simulink model "PhysicalHyperCook"  (R2026b)
settings: Solver=VariableStepAuto  StopTime=14400
undefined symbols (not defined in the file): Fault_T_Cook1, Fault_T_Cook2, Fault_T_Cook3, Fault_T_Cook4, Fault_T_Pack, Fault_T_Prep1, Fault_T_Prep2, Fault_T_QC, HC_PackRate_bph, HC_PrepRate_bph, HC_QCRate_bph, HC_Resupply_bph, Recipe_Block_s, Recipe_Count, Recipe_Flush_s, Resupply_Cutoff_T, Transport_Latency_s, Transport_Rate_bph
(part 1 of 2)
settings Model: DataDictionary=PhysicalHyperCookData.sldd  Creator=sarah  LastModifiedBy=sdagen

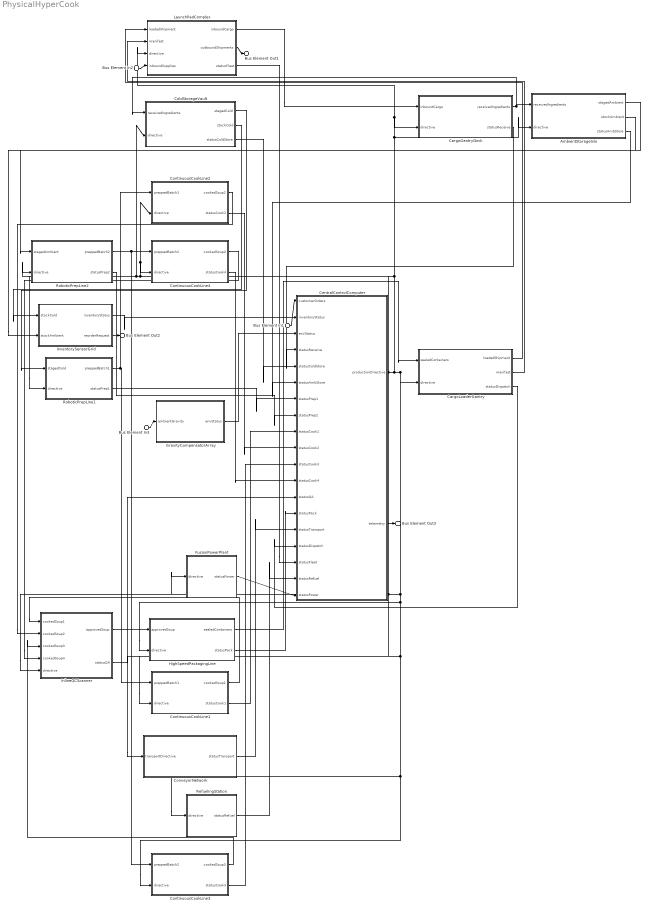
== system PhysicalHyperCook ==
  Bus Element In1 : Inport  PortName=CustomerOrders
  Bus Element In2 : Inport  Port=2  PortName=InboundSupplies
  Bus Element In3 : Inport  Port=3  PortName=AmbientGravity
  AmbientStorageSilo : Subsystem
      settings: PortSchema="{\"entries\":[{\"content\":{\"headerSize\":26,\"margin\":15,\"minimumSpacing\":25,\"sides\":[{\"content\":{\"connectorIds\":[\"In1\",\"In2\"]},\"type\":\"ConnectorPlacement.EquallySpacedRectSide\",\"uuid\":\"f830f98a-8e8b-4468-adf4-d6eab644987f\"},{\"content\":{\"connectorIds\":[\"Out1\",\"Out2\",\"Out3\"],\"side\":\"RIGHT\"},\"type\":\"ConnectorPlacement.EquallySpacedRectSide\",\"uuid\":\"7e0d0116-b3ba-4668-b638-30d0f54ba087\"},{\"content\":{\"side\":\"TOP\"},\"type\":\"ConnectorPlacement.EquallySpacedRectSide\",\"uuid\":\"7b4146d3-46d2-45ca-8c34-b106f0d8cedd\"}]},\"type\":\"ConnectorPlacement.EquallySpacedConnector\",\"uuid\":\"3d911b2d-a78f-42ea-b869-5e09982d9f54\"}],\"packageUris\":[\"http://schema.mathworks.com/mf0/Connector/R2020b\"],\"version\":\"1.0\"}"
  CargoGantryDock : Subsystem
      settings: PortSchema="{\"entries\":[{\"content\":{\"headerSize\":26,\"margin\":15,\"minimumSpacing\":25,\"sides\":[{\"content\":{\"connectorIds\":[\"In1\",\"In2\"]},\"type\":\"ConnectorPlacement.EquallySpacedRectSide\",\"uuid\":\"f830f98a-8e8b-4468-adf4-d6eab644987f\"},{\"content\":{\"connectorIds\":[\"Out1\",\"Out2\"],\"side\":\"RIGHT\"},\"type\":\"ConnectorPlacement.EquallySpacedRectSide\",\"uuid\":\"7e0d0116-b3ba-4668-b638-30d0f54ba087\"},{\"content\":{\"side\":\"TOP\"},\"type\":\"ConnectorPlacement.EquallySpacedRectSide\",\"uuid\":\"7b4146d3-46d2-45ca-8c34-b106f0d8cedd\"}]},\"type\":\"ConnectorPlacement.EquallySpacedConnector\",\"uuid\":\"3d911b2d-a78f-42ea-b869-5e09982d9f54\"}],\"packageUris\":[\"http://schema.mathworks.com/mf0/Connector/R2020b\"],\"version\":\"1.0\"}"
  CargoLoaderGantry : Subsystem
      settings: PortSchema="{\"entries\":[{\"content\":{\"headerSize\":26,\"margin\":15,\"minimumSpacing\":25,\"sides\":[{\"content\":{\"connectorIds\":[\"In1\",\"In2\"]},\"type\":\"ConnectorPlacement.EquallySpacedRectSide\",\"uuid\":\"f830f98a-8e8b-4468-adf4-d6eab644987f\"},{\"content\":{\"connectorIds\":[\"Out1\",\"Out2\",\"Out3\"],\"side\":\"RIGHT\"},\"type\":\"ConnectorPlacement.EquallySpacedRectSide\",\"uuid\":\"7e0d0116-b3ba-4668-b638-30d0f54ba087\"},{\"content\":{\"side\":\"TOP\"},\"type\":\"ConnectorPlacement.EquallySpacedRectSide\",\"uuid\":\"7b4146d3-46d2-45ca-8c34-b106f0d8cedd\"}]},\"type\":\"ConnectorPlacement.EquallySpacedConnector\",\"uuid\":\"3d911b2d-a78f-42ea-b869-5e09982d9f54\"}],\"packageUris\":[\"http://schema.mathworks.com/mf0/Connector/R2020b\"],\"version\":\"1.0\"}"
  CentralControlComputer : Subsystem
      settings: PortSchema="{\"entries\":[{\"content\":{\"headerSize\":26,\"margin\":15,\"minimumSpacing\":25,\"sides\":[{\"content\":{\"connectorIds\":[\"In1\",\"In2\",\"In3\",\"In4\",\"In5\",\"In6\",\"In7\",\"In8\",\"In9\",\"In10\",\"In11\",\"In12\",\"In13\",\"In14\",\"In15\",\"In16\",\"In17\",\"In18\",\"In19\"]},\"type\":\"ConnectorPlacement.EquallySpacedRectSide\",\"uuid\":\"f830f98a-8e8b-4468-adf4-d6eab644987f\"},{\"content\":{\"connectorIds\":[\"Out1\",\"Out2\"],\"side\":\"RIGHT\"},\"type\":\"ConnectorPlacement.EquallySpacedRectSide\",\"uuid\":\"7e0d0116-b3ba-4668-b638-30d0f54ba087\"},{\"content\":{\"side\":\"TOP\"},\"type\":\"ConnectorPlacement.EquallySpacedRectSide\",\"uuid\":\"7b4146d3-46d2-45ca-8c34-b106f0d8cedd\"}]},\"type\":\"ConnectorPlacement.EquallySpacedConnector\",\"uuid\":\"3d911b2d-a78f-42ea-b869-5e09982d9f54\"}],\"packageUris\":[\"http://schema.mathworks.com/mf0/Connector/R2020b\"],\"version\":\"1.0\"}"
  ColdStorageVault : Subsystem
      settings: PortSchema="{\"entries\":[{\"content\":{\"headerSize\":26,\"margin\":15,\"minimumSpacing\":25,\"sides\":[{\"content\":{\"connectorIds\":[\"In1\",\"In2\"]},\"type\":\"ConnectorPlacement.EquallySpacedRectSide\",\"uuid\":\"f830f98a-8e8b-4468-adf4-d6eab644987f\"},{\"content\":{\"connectorIds\":[\"Out1\",\"Out2\",\"Out3\"],\"side\":\"RIGHT\"},\"type\":\"ConnectorPlacement.EquallySpacedRectSide\",\"uuid\":\"7e0d0116-b3ba-4668-b638-30d0f54ba087\"},{\"content\":{\"side\":\"TOP\"},\"type\":\"ConnectorPlacement.EquallySpacedRectSide\",\"uuid\":\"7b4146d3-46d2-45ca-8c34-b106f0d8cedd\"}]},\"type\":\"ConnectorPlacement.EquallySpacedConnector\",\"uuid\":\"3d911b2d-a78f-42ea-b869-5e09982d9f54\"}],\"packageUris\":[\"http://schema.mathworks.com/mf0/Connector/R2020b\"],\"version\":\"1.0\"}"
  ContinuousCookLine1 : Subsystem
      settings: PortSchema="{\"entries\":[{\"content\":{\"headerSize\":26,\"margin\":15,\"minimumSpacing\":25,\"sides\":[{\"content\":{\"connectorIds\":[\"In1\",\"In2\"]},\"type\":\"ConnectorPlacement.EquallySpacedRectSide\",\"uuid\":\"f830f98a-8e8b-4468-adf4-d6eab644987f\"},{\"content\":{\"connectorIds\":[\"Out1\",\"Out2\"],\"side\":\"RIGHT\"},\"type\":\"ConnectorPlacement.EquallySpacedRectSide\",\"uuid\":\"7e0d0116-b3ba-4668-b638-30d0f54ba087\"},{\"content\":{\"side\":\"TOP\"},\"type\":\"ConnectorPlacement.EquallySpacedRectSide\",\"uuid\":\"7b4146d3-46d2-45ca-8c34-b106f0d8cedd\"}]},\"type\":\"ConnectorPlacement.EquallySpacedConnector\",\"uuid\":\"3d911b2d-a78f-42ea-b869-5e09982d9f54\"}],\"packageUris\":[\"http://schema.mathworks.com/mf0/Connector/R2020b\"],\"version\":\"1.0\"}"
  ContinuousCookLine2 : Subsystem
      settings: PortSchema="{\"entries\":[{\"content\":{\"headerSize\":26,\"margin\":15,\"minimumSpacing\":25,\"sides\":[{\"content\":{\"connectorIds\":[\"In1\",\"In2\"]},\"type\":\"ConnectorPlacement.EquallySpacedRectSide\",\"uuid\":\"f830f98a-8e8b-4468-adf4-d6eab644987f\"},{\"content\":{\"connectorIds\":[\"Out1\",\"Out2\"],\"side\":\"RIGHT\"},\"type\":\"ConnectorPlacement.EquallySpacedRectSide\",\"uuid\":\"7e0d0116-b3ba-4668-b638-30d0f54ba087\"},{\"content\":{\"side\":\"TOP\"},\"type\":\"ConnectorPlacement.EquallySpacedRectSide\",\"uuid\":\"7b4146d3-46d2-45ca-8c34-b106f0d8cedd\"}]},\"type\":\"ConnectorPlacement.EquallySpacedConnector\",\"uuid\":\"3d911b2d-a78f-42ea-b869-5e09982d9f54\"}],\"packageUris\":[\"http://schema.mathworks.com/mf0/Connector/R2020b\"],\"version\":\"1.0\"}"
  ContinuousCookLine3 : Subsystem
      settings: PortSchema="{\"entries\":[{\"content\":{\"headerSize\":26,\"margin\":15,\"minimumSpacing\":25,\"sides\":[{\"content\":{\"connectorIds\":[\"In1\",\"In2\"]},\"type\":\"ConnectorPlacement.EquallySpacedRectSide\",\"uuid\":\"f830f98a-8e8b-4468-adf4-d6eab644987f\"},{\"content\":{\"connectorIds\":[\"Out1\",\"Out2\"],\"side\":\"RIGHT\"},\"type\":\"ConnectorPlacement.EquallySpacedRectSide\",\"uuid\":\"7e0d0116-b3ba-4668-b638-30d0f54ba087\"},{\"content\":{\"side\":\"TOP\"},\"type\":\"ConnectorPlacement.EquallySpacedRectSide\",\"uuid\":\"7b4146d3-46d2-45ca-8c34-b106f0d8cedd\"}]},\"type\":\"ConnectorPlacement.EquallySpacedConnector\",\"uuid\":\"3d911b2d-a78f-42ea-b869-5e09982d9f54\"}],\"packageUris\":[\"http://schema.mathworks.com/mf0/Connector/R2020b\"],\"version\":\"1.0\"}"
  ContinuousCookLine4 : Subsystem
      settings: PortSchema="{\"entries\":[{\"content\":{\"headerSize\":26,\"margin\":15,\"minimumSpacing\":25,\"sides\":[{\"content\":{\"connectorIds\":[\"In1\",\"In2\"]},\"type\":\"ConnectorPlacement.EquallySpacedRectSide\",\"uuid\":\"f830f98a-8e8b-4468-adf4-d6eab644987f\"},{\"content\":{\"connectorIds\":[\"Out1\",\"Out2\"],\"side\":\"RIGHT\"},\"type\":\"ConnectorPlacement.EquallySpacedRectSide\",\"uuid\":\"7e0d0116-b3ba-4668-b638-30d0f54ba087\"},{\"content\":{\"side\":\"TOP\"},\"type\":\"ConnectorPlacement.EquallySpacedRectSide\",\"uuid\":\"7b4146d3-46d2-45ca-8c34-b106f0d8cedd\"}]},\"type\":\"ConnectorPlacement.EquallySpacedConnector\",\"uuid\":\"3d911b2d-a78f-42ea-b869-5e09982d9f54\"}],\"packageUris\":[\"http://schema.mathworks.com/mf0/Connector/R2020b\"],\"version\":\"1.0\"}"
  ConveyorNetwork : Subsystem
      settings: PortSchema="{\"entries\":[{\"content\":{\"headerSize\":26,\"margin\":15,\"minimumSpacing\":25,\"sides\":[{\"content\":{\"connectorIds\":[\"In1\"]},\"type\":\"ConnectorPlacement.EquallySpacedRectSide\",\"uuid\":\"f830f98a-8e8b-4468-adf4-d6eab644987f\"},{\"content\":{\"connectorIds\":[\"Out1\"],\"side\":\"RIGHT\"},\"type\":\"ConnectorPlacement.EquallySpacedRectSide\",\"uuid\":\"7e0d0116-b3ba-4668-b638-30d0f54ba087\"},{\"content\":{\"side\":\"TOP\"},\"type\":\"ConnectorPlacement.EquallySpacedRectSide\",\"uuid\":\"7b4146d3-46d2-45ca-8c34-b106f0d8cedd\"}]},\"type\":\"ConnectorPlacement.EquallySpacedConnector\",\"uuid\":\"3d911b2d-a78f-42ea-b869-5e09982d9f54\"}],\"packageUris\":[\"http://schema.mathworks.com/mf0/Connector/R2020b\"],\"version\":\"1.0\"}"
  FusionPowerPlant : Subsystem
      settings: PortSchema="{\"entries\":[{\"content\":{\"headerSize\":26,\"margin\":15,\"minimumSpacing\":25,\"sides\":[{\"content\":{\"connectorIds\":[\"In1\"]},\"type\":\"ConnectorPlacement.EquallySpacedRectSide\",\"uuid\":\"f830f98a-8e8b-4468-adf4-d6eab644987f\"},{\"content\":{\"connectorIds\":[\"Out1\"],\"side\":\"RIGHT\"},\"type\":\"ConnectorPlacement.EquallySpacedRectSide\",\"uuid\":\"7e0d0116-b3ba-4668-b638-30d0f54ba087\"},{\"content\":{\"side\":\"TOP\"},\"type\":\"ConnectorPlacement.EquallySpacedRectSide\",\"uuid\":\"7b4146d3-46d2-45ca-8c34-b106f0d8cedd\"}]},\"type\":\"ConnectorPlacement.EquallySpacedConnector\",\"uuid\":\"3d911b2d-a78f-42ea-b869-5e09982d9f54\"}],\"packageUris\":[\"http://schema.mathworks.com/mf0/Connector/R2020b\"],\"version\":\"1.0\"}"
  GravityCompensatorArray : Subsystem
      settings: PortSchema="{\"entries\":[{\"content\":{\"headerSize\":26,\"margin\":15,\"minimumSpacing\":25,\"sides\":[{\"content\":{\"connectorIds\":[\"In1\"]},\"type\":\"ConnectorPlacement.EquallySpacedRectSide\",\"uuid\":\"f830f98a-8e8b-4468-adf4-d6eab644987f\"},{\"content\":{\"connectorIds\":[\"Out1\"],\"side\":\"RIGHT\"},\"type\":\"ConnectorPlacement.EquallySpacedRectSide\",\"uuid\":\"7e0d0116-b3ba-4668-b638-30d0f54ba087\"},{\"content\":{\"side\":\"TOP\"},\"type\":\"ConnectorPlacement.EquallySpacedRectSide\",\"uuid\":\"7b4146d3-46d2-45ca-8c34-b106f0d8cedd\"}]},\"type\":\"ConnectorPlacement.EquallySpacedConnector\",\"uuid\":\"3d911b2d-a78f-42ea-b869-5e09982d9f54\"}],\"packageUris\":[\"http://schema.mathworks.com/mf0/Connector/R2020b\"],\"version\":\"1.0\"}"
  HighSpeedPackagingLine : Subsystem
      settings: PortSchema="{\"entries\":[{\"content\":{\"headerSize\":26,\"margin\":15,\"minimumSpacing\":25,\"sides\":[{\"content\":{\"connectorIds\":[\"In1\",\"In2\"]},\"type\":\"ConnectorPlacement.EquallySpacedRectSide\",\"uuid\":\"f830f98a-8e8b-4468-adf4-d6eab644987f\"},{\"content\":{\"connectorIds\":[\"Out1\",\"Out2\"],\"side\":\"RIGHT\"},\"type\":\"ConnectorPlacement.EquallySpacedRectSide\",\"uuid\":\"7e0d0116-b3ba-4668-b638-30d0f54ba087\"},{\"content\":{\"side\":\"TOP\"},\"type\":\"ConnectorPlacement.EquallySpacedRectSide\",\"uuid\":\"7b4146d3-46d2-45ca-8c34-b106f0d8cedd\"}]},\"type\":\"ConnectorPlacement.EquallySpacedConnector\",\"uuid\":\"3d911b2d-a78f-42ea-b869-5e09982d9f54\"}],\"packageUris\":[\"http://schema.mathworks.com/mf0/Connector/R2020b\"],\"version\":\"1.0\"}"
  InlineQCScanner : Subsystem
      settings: PortSchema="{\"entries\":[{\"content\":{\"headerSize\":26,\"margin\":15,\"minimumSpacing\":25,\"sides\":[{\"content\":{\"connectorIds\":[\"In1\",\"In2\",\"In3\",\"In4\",\"In5\"]},\"type\":\"ConnectorPlacement.EquallySpacedRectSide\",\"uuid\":\"f830f98a-8e8b-4468-adf4-d6eab644987f\"},{\"content\":{\"connectorIds\":[\"Out1\",\"Out2\"],\"side\":\"RIGHT\"},\"type\":\"ConnectorPlacement.EquallySpacedRectSide\",\"uuid\":\"7e0d0116-b3ba-4668-b638-30d0f54ba087\"},{\"content\":{\"side\":\"TOP\"},\"type\":\"ConnectorPlacement.EquallySpacedRectSide\",\"uuid\":\"7b4146d3-46d2-45ca-8c34-b106f0d8cedd\"}]},\"type\":\"ConnectorPlacement.EquallySpacedConnector\",\"uuid\":\"3d911b2d-a78f-42ea-b869-5e09982d9f54\"}],\"packageUris\":[\"http://schema.mathworks.com/mf0/Connector/R2020b\"],\"version\":\"1.0\"}"
  InventorySensorGrid : Subsystem
      settings: PortSchema="{\"entries\":[{\"content\":{\"headerSize\":26,\"margin\":15,\"minimumSpacing\":25,\"sides\":[{\"content\":{\"connectorIds\":[\"In1\",\"In2\"]},\"type\":\"ConnectorPlacement.EquallySpacedRectSide\",\"uuid\":\"f830f98a-8e8b-4468-adf4-d6eab644987f\"},{\"content\":{\"connectorIds\":[\"Out1\",\"Out2\"],\"side\":\"RIGHT\"},\"type\":\"ConnectorPlacement.EquallySpacedRectSide\",\"uuid\":\"7e0d0116-b3ba-4668-b638-30d0f54ba087\"},{\"content\":{\"side\":\"TOP\"},\"type\":\"ConnectorPlacement.EquallySpacedRectSide\",\"uuid\":\"7b4146d3-46d2-45ca-8c34-b106f0d8cedd\"}]},\"type\":\"ConnectorPlacement.EquallySpacedConnector\",\"uuid\":\"3d911b2d-a78f-42ea-b869-5e09982d9f54\"}],\"packageUris\":[\"http://schema.mathworks.com/mf0/Connector/R2020b\"],\"version\":\"1.0\"}"
  LaunchPadComplex : Subsystem
      settings: PortSchema="{\"entries\":[{\"content\":{\"headerSize\":26,\"margin\":15,\"minimumSpacing\":25,\"sides\":[{\"content\":{\"connectorIds\":[\"In1\",\"In2\",\"In3\",\"In4\"]},\"type\":\"ConnectorPlacement.EquallySpacedRectSide\",\"uuid\":\"f830f98a-8e8b-4468-adf4-d6eab644987f\"},{\"content\":{\"connectorIds\":[\"Out1\",\"Out2\",\"Out3\"],\"side\":\"RIGHT\"},\"type\":\"ConnectorPlacement.EquallySpacedRectSide\",\"uuid\":\"7e0d0116-b3ba-4668-b638-30d0f54ba087\"},{\"content\":{\"side\":\"TOP\"},\"type\":\"ConnectorPlacement.EquallySpacedRectSide\",\"uuid\":\"7b4146d3-46d2-45ca-8c34-b106f0d8cedd\"}]},\"type\":\"ConnectorPlacement.EquallySpacedConnector\",\"uuid\":\"3d911b2d-a78f-42ea-b869-5e09982d9f54\"}],\"packageUris\":[\"http://schema.mathworks.com/mf0/Connector/R2020b\"],\"version\":\"1.0\"}"
  RefuelingStation : Subsystem
      settings: PortSchema="{\"entries\":[{\"content\":{\"headerSize\":26,\"margin\":15,\"minimumSpacing\":25,\"sides\":[{\"content\":{\"connectorIds\":[\"In1\"]},\"type\":\"ConnectorPlacement.EquallySpacedRectSide\",\"uuid\":\"f830f98a-8e8b-4468-adf4-d6eab644987f\"},{\"content\":{\"connectorIds\":[\"Out1\"],\"side\":\"RIGHT\"},\"type\":\"ConnectorPlacement.EquallySpacedRectSide\",\"uuid\":\"7e0d0116-b3ba-4668-b638-30d0f54ba087\"},{\"content\":{\"side\":\"TOP\"},\"type\":\"ConnectorPlacement.EquallySpacedRectSide\",\"uuid\":\"7b4146d3-46d2-45ca-8c34-b106f0d8cedd\"}]},\"type\":\"ConnectorPlacement.EquallySpacedConnector\",\"uuid\":\"3d911b2d-a78f-42ea-b869-5e09982d9f54\"}],\"packageUris\":[\"http://schema.mathworks.com/mf0/Connector/R2020b\"],\"version\":\"1.0\"}"
  RoboticPrepLine1 : Subsystem
      settings: PortSchema="{\"entries\":[{\"content\":{\"headerSize\":26,\"margin\":15,\"minimumSpacing\":25,\"sides\":[{\"content\":{\"connectorIds\":[\"In1\",\"In2\"]},\"type\":\"ConnectorPlacement.EquallySpacedRectSide\",\"uuid\":\"f830f98a-8e8b-4468-adf4-d6eab644987f\"},{\"content\":{\"connectorIds\":[\"Out1\",\"Out2\"],\"side\":\"RIGHT\"},\"type\":\"ConnectorPlacement.EquallySpacedRectSide\",\"uuid\":\"7e0d0116-b3ba-4668-b638-30d0f54ba087\"},{\"content\":{\"side\":\"TOP\"},\"type\":\"ConnectorPlacement.EquallySpacedRectSide\",\"uuid\":\"7b4146d3-46d2-45ca-8c34-b106f0d8cedd\"}]},\"type\":\"ConnectorPlacement.EquallySpacedConnector\",\"uuid\":\"3d911b2d-a78f-42ea-b869-5e09982d9f54\"}],\"packageUris\":[\"http://schema.mathworks.com/mf0/Connector/R2020b\"],\"version\":\"1.0\"}"
  RoboticPrepLine2 : Subsystem
      settings: PortSchema="{\"entries\":[{\"content\":{\"headerSize\":26,\"margin\":15,\"minimumSpacing\":25,\"sides\":[{\"content\":{\"connectorIds\":[\"In1\",\"In2\"]},\"type\":\"ConnectorPlacement.EquallySpacedRectSide\",\"uuid\":\"f830f98a-8e8b-4468-adf4-d6eab644987f\"},{\"content\":{\"connectorIds\":[\"Out1\",\"Out2\"],\"side\":\"RIGHT\"},\"type\":\"ConnectorPlacement.EquallySpacedRectSide\",\"uuid\":\"7e0d0116-b3ba-4668-b638-30d0f54ba087\"},{\"content\":{\"side\":\"TOP\"},\"type\":\"ConnectorPlacement.EquallySpacedRectSide\",\"uuid\":\"7b4146d3-46d2-45ca-8c34-b106f0d8cedd\"}]},\"type\":\"ConnectorPlacement.EquallySpacedConnector\",\"uuid\":\"3d911b2d-a78f-42ea-b869-5e09982d9f54\"}],\"packageUris\":[\"http://schema.mathworks.com/mf0/Connector/R2020b\"],\"version\":\"1.0\"}"
  Bus Element Out1 : Outport  PortName=OutboundShipments
  Bus Element Out2 : Outport  Port=2  PortName=ReorderRequests
  Bus Element Out3 : Outport  Port=3  PortName=Telemetry
  wires:
  AmbientStorageSilo/1(stagedAmbient) -> RoboticPrepLine2/1(stagedAmbient)
  LaunchPadComplex/3(statusFleet) -> CentralControlComputer/17(statusFleet)
  Bus Element In2/1 -> LaunchPadComplex/4(inboundSupplies)
  Bus Element In3/1 -> GravityCompensatorArray/1(ambientGravity)
  RoboticPrepLine2/1(preppedBatch2) -> ContinuousCookLine4/1(preppedBatch2), ContinuousCookLine3/1(preppedBatch2)
  InventorySensorGrid/2(reorderRequest) -> Bus Element Out2/1
  InventorySensorGrid/1(inventoryStatus) -> CentralControlComputer/2(inventoryStatus)
  RoboticPrepLine2/2(statusPrep2) -> CentralControlComputer/8(statusPrep2)
  ColdStorageVault/2(stockCold) -> InventorySensorGrid/1(stockCold)
  RoboticPrepLine1/1(preppedBatch1) -> ContinuousCookLine2/1(preppedBatch1), ContinuousCookLine1/1(preppedBatch1)
  RefuelingStation/1(statusRefuel) -> CentralControlComputer/18(statusRefuel)
  RoboticPrepLine1/2(statusPrep1) -> CentralControlComputer/7(statusPrep1)
  ContinuousCookLine4/1(cookedSoup4) -> InlineQCScanner/4(cookedSoup4)
  InlineQCScanner/1(approvedSoup) -> HighSpeedPackagingLine/1(approvedSoup)
  InlineQCScanner/2(statusQA) -> CentralControlComputer/13(statusQA)
  LaunchPadComplex/1(inboundCargo) -> CargoGantryDock/1(inboundCargo)
  CargoLoaderGantry/3(statusDispatch) -> CentralControlComputer/16(statusDispatch)
  LaunchPadComplex/2(outboundShipments) -> Bus Element Out1/1
  ColdStorageVault/1(stagedCold) -> RoboticPrepLine1/1(stagedCold)
  AmbientStorageSilo/3(statusAmbStore) -> CentralControlComputer/6(statusAmbStore)
  ColdStorageVault/3(statusColdStore) -> CentralControlComputer/5(statusColdStore)
  ContinuousCookLine3/1(cookedSoup3) -> InlineQCScanner/3(cookedSoup3)
  FusionPowerPlant/1(statusPower) -> CentralControlComputer/19(statusPower)
  ContinuousCookLine2/1(cookedSoup2) -> InlineQCScanner/2(cookedSoup2)
  ContinuousCookLine2/2(statusCook2) -> CentralControlComputer/10(statusCook2)
  ContinuousCookLine4/2(statusCook4) -> CentralControlComputer/12(statusCook4)
  Bus Element In1/1 -> CentralControlComputer/1(customerOrders)
  GravityCompensatorArray/1(envStatus) -> CentralControlComputer/3(envStatus)
  HighSpeedPackagingLine/1(sealedContainers) -> CargoLoaderGantry/1(sealedContainers)
  HighSpeedPackagingLine/2(statusPack) -> CentralControlComputer/14(statusPack)
  ContinuousCookLine1/1(cookedSoup1) -> InlineQCScanner/1(cookedSoup1)
  CentralControlComputer/2(telemetry) -> Bus Element Out3/1
  ContinuousCookLine1/2(statusCook1) -> CentralControlComputer/9(statusCook1)
  ConveyorNetwork/1(statusTransport) -> CentralControlComputer/15(statusTransport)
  ContinuousCookLine3/2(statusCook3) -> CentralControlComputer/11(statusCook3)
  CentralControlComputer/1(productionDirective) -> ContinuousCookLine1/2(directive), FusionPowerPlant/1(directive), ContinuousCookLine3/2(directive), RefuelingStation/1(directive), ConveyorNetwork/1(transportDirective), HighSpeedPackagingLine/2(directive), InlineQCScanner/5(directive), CargoLoaderGantry/2(directive), RoboticPrepLine2/2(directive), ColdStorageVault/2(directive), ContinuousCookLine4/2(directive), ContinuousCookLine2/2(directive), LaunchPadComplex/3(directive), CargoGantryDock/2(directive), AmbientStorageSilo/2(directive), RoboticPrepLine1/2(directive)
  CargoGantryDock/1(receivedIngredients) -> ColdStorageVault/1(receivedIngredients), AmbientStorageSilo/1(receivedIngredients)
  CargoGantryDock/2(statusReceive) -> CentralControlComputer/4(statusReceive)
  CargoLoaderGantry/1(loadedShipment) -> LaunchPadComplex/1(loadedShipment)
  CargoLoaderGantry/2(manifest) -> LaunchPadComplex/2(manifest)
  AmbientStorageSilo/2(stockAmbient) -> InventorySensorGrid/2(stockAmbient)

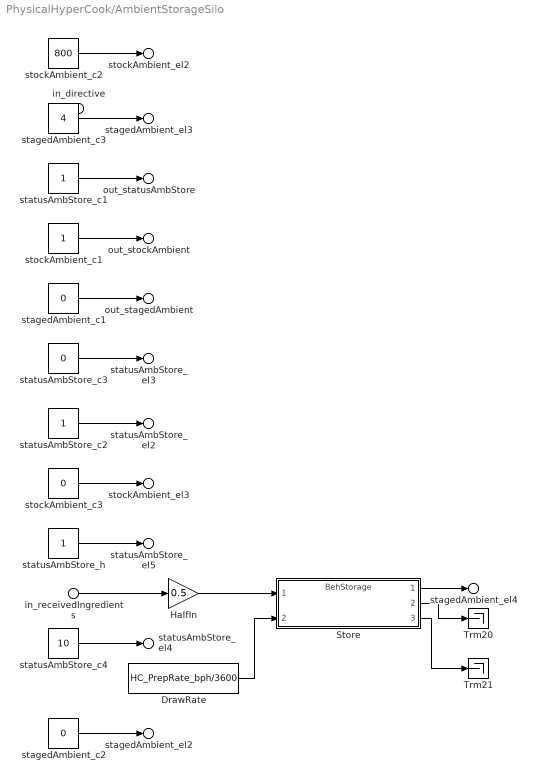
== system PhysicalHyperCook/AmbientStorageSilo ==
  in_receivedIngredients : Inport  PortName=receivedIngredients  Element=flow_bps
  in_directive : Inport  Port=2  PortName=directive  Element=setpoint
  DrawRate : Constant  Value=HC_PrepRate_bph/3600
  HalfIn : Gain  Gain=0.5
  Store : ModelReference  ModelNameDialog=BehStorage  UsingDefaultArgumentValue=0,0  SimulationMode=Normal  ModelReferenceVersion=1.4
  Trm20 : Terminator
  Trm21 : Terminator
  stagedAmbient_c1 : Constant  Value=0
  stagedAmbient_c2 : Constant  Value=0
  stagedAmbient_c3 : Constant  Value=4
  statusAmbStore_c1 : Constant
  statusAmbStore_c2 : Constant
  statusAmbStore_c3 : Constant  Value=0
  statusAmbStore_c4 : Constant  Value=10
  statusAmbStore_h : Constant
  stockAmbient_c1 : Constant
  stockAmbient_c2 : Constant  Value=800
  stockAmbient_c3 : Constant  Value=0
  out_stagedAmbient : Outport  PortName=stagedAmbient  Element=palletId
  stagedAmbient_el2 : Outport  PortName=stagedAmbient  Element=mass_kg
  stagedAmbient_el3 : Outport  PortName=stagedAmbient  Element=temp_C
  stagedAmbient_el4 : Outport  PortName=stagedAmbient  Element=flow_bps
  out_stockAmbient : Outport  Port=2  PortName=stockAmbient  Element=itemId
  stockAmbient_el2 : Outport  Port=2  PortName=stockAmbient  Element=qty_units
  stockAmbient_el3 : Outport  Port=2  PortName=stockAmbient  Element=error_pct
  out_statusAmbStore : Outport  Port=3  PortName=statusAmbStore  Element=unitId
  statusAmbStore_el2 : Outport  Port=3  PortName=statusAmbStore  Element=opState
  statusAmbStore_el3 : Outport  Port=3  PortName=statusAmbStore  Element=faultCode
  statusAmbStore_el4 : Outport  Port=3  PortName=statusAmbStore  Element=power_kW
  statusAmbStore_el5 : Outport  Port=3  PortName=statusAmbStore  Element=health
  wires:
  stockAmbient_c2/1 -> stockAmbient_el2/1
  stagedAmbient_c3/1 -> stagedAmbient_el3/1
  statusAmbStore_c1/1 -> out_statusAmbStore/1
  stockAmbient_c3/1 -> stockAmbient_el3/1
  stockAmbient_c1/1 -> out_stockAmbient/1
  stagedAmbient_c1/1 -> out_stagedAmbient/1
  statusAmbStore_c3/1 -> statusAmbStore_el3/1
  statusAmbStore_c2/1 -> statusAmbStore_el2/1
  statusAmbStore_h/1 -> statusAmbStore_el5/1
  in_receivedIngredients/1 -> HalfIn/1
  statusAmbStore_c4/1 -> statusAmbStore_el4/1
  stagedAmbient_c2/1 -> stagedAmbient_el2/1
  HalfIn/1 -> Store/1
  DrawRate/1 -> Store/2
  Store/1 -> stagedAmbient_el4/1
  Store/2 -> Trm20/1
  Store/3 -> Trm21/1

== system PhysicalHyperCook/CargoGantryDock ==
  in_inboundCargo : Inport  PortName=inboundCargo  Element=flow_bps
  in_directive : Inport  Port=2  PortName=directive
  in_inboundCargoCap : Saturate  UpperLimit=0.111111111111  LowerLimit=0
  receivedIngredients_c1 : Constant  Value=0
  receivedIngredients_c2 : Constant  Value=0
  receivedIngredients_c3 : Constant  Value=4
  statusReceive_c1 : Constant
  statusReceive_c2 : Constant
  statusReceive_c3 : Constant  Value=0
  statusReceive_c4 : Constant  Value=15
  statusReceive_h : Constant
  out_receivedIngredients : Outport  PortName=receivedIngredients  Element=palletId
  receivedIngredients_el2 : Outport  PortName=receivedIngredients  Element=mass_kg
  receivedIngredients_el3 : Outport  PortName=receivedIngredients  Element=temp_C
  receivedIngredients_el4 : Outport  PortName=receivedIngredients  Element=flow_bps
  out_statusReceive : Outport  Port=2  PortName=statusReceive  Element=unitId
  statusReceive_el2 : Outport  Port=2  PortName=statusReceive  Element=opState
  statusReceive_el3 : Outport  Port=2  PortName=statusReceive  Element=faultCode
  statusReceive_el4 : Outport  Port=2  PortName=statusReceive  Element=power_kW
  statusReceive_el5 : Outport  Port=2  PortName=statusReceive  Element=health
  wires:
  receivedIngredients_c3/1 -> receivedIngredients_el3/1
  statusReceive_c1/1 -> out_statusReceive/1
  statusReceive_h/1 -> statusReceive_el5/1
  statusReceive_c4/1 -> statusReceive_el4/1
  receivedIngredients_c2/1 -> receivedIngredients_el2/1
  statusReceive_c2/1 -> statusReceive_el2/1
  in_inboundCargo/1 -> in_inboundCargoCap/1
  receivedIngredients_c1/1 -> out_receivedIngredients/1
  in_inboundCargoCap/1 -> receivedIngredients_el4/1
  statusReceive_c3/1 -> statusReceive_el3/1

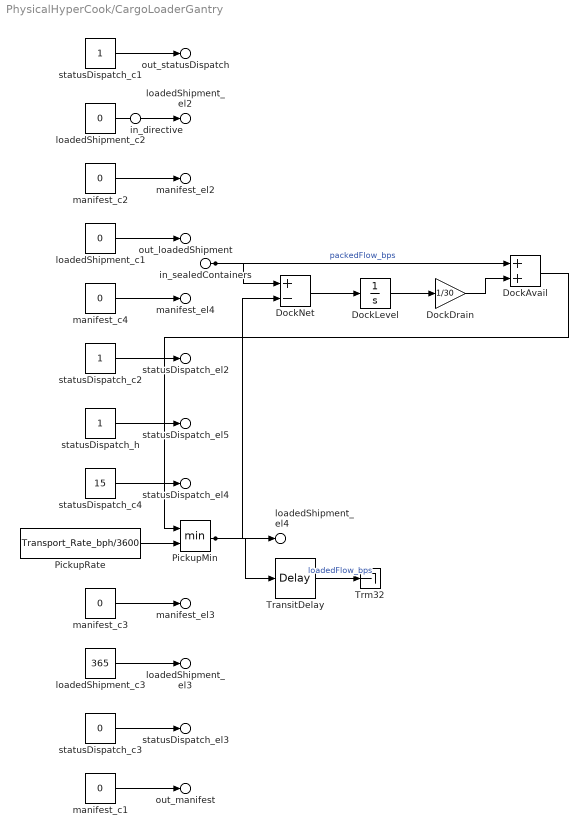
== system PhysicalHyperCook/CargoLoaderGantry ==
  in_sealedContainers : Inport  PortName=sealedContainers  Element=flow_bps
  in_directive : Inport  Port=2  PortName=directive
  DockAvail : Sum
  DockDrain : Gain  Gain=1/30
  DockLevel : Integrator  LimitOutput=on  UpperSaturationLimit=600  LowerSaturationLimit=0
  DockNet : Sum  Inputs=+-
  PickupMin : MinMax  Inputs=2
  PickupRate : Constant  Value=Transport_Rate_bph/3600
  TransitDelay : TransportDelay  DelayTime=Transport_Latency_s
  Trm32 : Terminator
  loadedShipment_c1 : Constant  Value=0
  loadedShipment_c2 : Constant  Value=0
  loadedShipment_c3 : Constant  Value=365
  manifest_c{1..4} (4 alike) : Constant  Value=0
  statusDispatch_c1 : Constant
  statusDispatch_c2 : Constant
  statusDispatch_c3 : Constant  Value=0
  statusDispatch_c4 : Constant  Value=15
  statusDispatch_h : Constant
  out_loadedShipment : Outport  PortName=loadedShipment  Element=batchId
  loadedShipment_el2 : Outport  PortName=loadedShipment  Element=count
  loadedShipment_el3 : Outport  PortName=loadedShipment  Element=sealRating_days
  loadedShipment_el4 : Outport  PortName=loadedShipment  Element=flow_bps
  out_manifest : Outport  Port=2  PortName=manifest  Element=destinationId
  manifest_el2 : Outport  Port=2  PortName=manifest  Element=batchId
  manifest_el3 : Outport  Port=2  PortName=manifest  Element=count
  manifest_el4 : Outport  Port=2  PortName=manifest  Element=mass_kg
  out_statusDispatch : Outport  Port=3  PortName=statusDispatch  Element=unitId
  statusDispatch_el2 : Outport  Port=3  PortName=statusDispatch  Element=opState
  statusDispatch_el3 : Outport  Port=3  PortName=statusDispatch  Element=faultCode
  statusDispatch_el4 : Outport  Port=3  PortName=statusDispatch  Element=power_kW
  statusDispatch_el5 : Outport  Port=3  PortName=statusDispatch  Element=health
  wires:
  statusDispatch_c1/1 -> out_statusDispatch/1
  DockLevel/1 -> DockDrain/1
  statusDispatch_c4/1 -> statusDispatch_el4/1
  loadedShipment_c2/1 -> loadedShipment_el2/1
  manifest_c2/1 -> manifest_el2/1
  loadedShipment_c1/1 -> out_loadedShipment/1
  manifest_c4/1 -> manifest_el4/1
  statusDispatch_c2/1 -> statusDispatch_el2/1
  statusDispatch_h/1 -> statusDispatch_el5/1
  PickupRate/1 -> PickupMin/2
  manifest_c3/1 -> manifest_el3/1
  loadedShipment_c3/1 -> loadedShipment_el3/1
  statusDispatch_c3/1 -> statusDispatch_el3/1
  manifest_c1/1 -> out_manifest/1
  in_sealedContainers/1 -> DockAvail/1, DockNet/1  "packedFlow_bps"
  PickupMin/1 -> DockNet/2, loadedShipment_el4/1, TransitDelay/1
  DockNet/1 -> DockLevel/1
  TransitDelay/1 -> Trm32/1  "loadedFlow_bps"
  DockDrain/1 -> DockAvail/2
  DockAvail/1 -> PickupMin/1

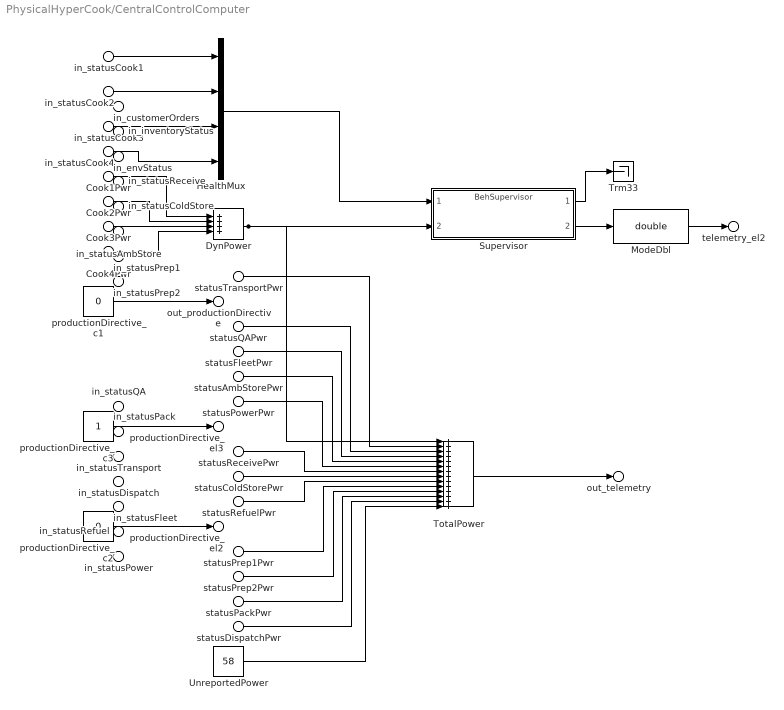
== system PhysicalHyperCook/CentralControlComputer ==
  in_customerOrders : Inport  PortName=customerOrders
  in_inventoryStatus : Inport  Port=2  PortName=inventoryStatus
  in_envStatus : Inport  Port=3  PortName=envStatus
  in_statusReceive : Inport  Port=4  PortName=statusReceive
  statusReceivePwr : Inport  Port=4  PortName=statusReceive  Element=power_kW
  in_statusColdStore : Inport  Port=5  PortName=statusColdStore
  statusColdStorePwr : Inport  Port=5  PortName=statusColdStore  Element=power_kW
  in_statusAmbStore : Inport  Port=6  PortName=statusAmbStore
  statusAmbStorePwr : Inport  Port=6  PortName=statusAmbStore  Element=power_kW
  in_statusPrep1 : Inport  Port=7  PortName=statusPrep1
  statusPrep1Pwr : Inport  Port=7  PortName=statusPrep1  Element=power_kW
  in_statusPrep2 : Inport  Port=8  PortName=statusPrep2
  statusPrep2Pwr : Inport  Port=8  PortName=statusPrep2  Element=power_kW
  Cook1Pwr : Inport  Port=9  PortName=statusCook1  Element=power_kW
  in_statusCook1 : Inport  Port=9  PortName=statusCook1  Element=health
  Cook2Pwr : Inport  Port=10  PortName=statusCook2  Element=power_kW
  in_statusCook2 : Inport  Port=10  PortName=statusCook2  Element=health
  Cook3Pwr : Inport  Port=11  PortName=statusCook3  Element=power_kW
  in_statusCook3 : Inport  Port=11  PortName=statusCook3  Element=health
  Cook4Pwr : Inport  Port=12  PortName=statusCook4  Element=power_kW
  in_statusCook4 : Inport  Port=12  PortName=statusCook4  Element=health
  in_statusQA : Inport  Port=13  PortName=statusQA
  statusQAPwr : Inport  Port=13  PortName=statusQA  Element=power_kW
  in_statusPack : Inport  Port=14  PortName=statusPack
  statusPackPwr : Inport  Port=14  PortName=statusPack  Element=power_kW
  in_statusTransport : Inport  Port=15  PortName=statusTransport
  statusTransportPwr : Inport  Port=15  PortName=statusTransport  Element=power_kW
  in_statusDispatch : Inport  Port=16  PortName=statusDispatch
  statusDispatchPwr : Inport  Port=16  PortName=statusDispatch  Element=power_kW
  in_statusFleet : Inport  Port=17  PortName=statusFleet
  statusFleetPwr : Inport  Port=17  PortName=statusFleet  Element=power_kW
  in_statusRefuel : Inport  Port=18  PortName=statusRefuel
  statusRefuelPwr : Inport  Port=18  PortName=statusRefuel  Element=power_kW
  in_statusPower : Inport  Port=19  PortName=statusPower
  statusPowerPwr : Inport  Port=19  PortName=statusPower  Element=power_kW
  DynPower : Sum  Inputs=++++
  HealthMux : Mux
  ModeDbl : DataTypeConversion  OutDataTypeStr=double  SaturateOnIntegerOverflow=off  RndMeth=Floor
  Supervisor : ModelReference  ModelNameDialog=BehSupervisor  ParameterArgumentNames=NumLines  ParameterArgumentValues=HC_NumLines  UsingDefaultArgumentValue=0  SimulationMode=Normal  ModelReferenceVersion=1.7
  TotalPower : Sum  Inputs=++++++++++++++
  Trm33 : Terminator
  UnreportedPower : Constant  Value=58
  productionDirective_c1 : Constant  Value=0
  productionDirective_c2 : Constant  Value=0
  productionDirective_c3 : Constant
  out_productionDirective : Outport  PortName=productionDirective  Element=cmdType
  productionDirective_el2 : Outport  PortName=productionDirective  Element=targetId
  productionDirective_el3 : Outport  PortName=productionDirective  Element=setpoint
  out_telemetry : Outport  Port=2  PortName=telemetry  Element=totalPower_kW
  telemetry_el2 : Outport  Port=2  PortName=telemetry  Element=plantMode
  wires:
  in_statusCook1/1 -> HealthMux/1
  Cook3Pwr/1 -> DynPower/3
  Cook1Pwr/1 -> DynPower/1
  Cook4Pwr/1 -> DynPower/4
  statusRefuelPwr/1 -> TotalPower/9
  in_statusCook2/1 -> HealthMux/2
  in_statusCook3/1 -> HealthMux/3
  in_statusCook4/1 -> HealthMux/4
  UnreportedPower/1 -> TotalPower/14
  statusAmbStorePwr/1 -> TotalPower/5
  Cook2Pwr/1 -> DynPower/2
  productionDirective_c1/1 -> out_productionDirective/1
  productionDirective_c3/1 -> productionDirective_el3/1
  productionDirective_c2/1 -> productionDirective_el2/1
  Supervisor/2 -> ModeDbl/1
  HealthMux/1 -> Supervisor/1
  statusFleetPwr/1 -> TotalPower/4
  DynPower/1 -> Supervisor/2, TotalPower/1
  statusTransportPwr/1 -> TotalPower/2
  statusQAPwr/1 -> TotalPower/3
  statusPowerPwr/1 -> TotalPower/6
  statusReceivePwr/1 -> TotalPower/7
  statusPackPwr/1 -> TotalPower/12
  statusColdStorePwr/1 -> TotalPower/8
  statusPrep1Pwr/1 -> TotalPower/10
  statusPrep2Pwr/1 -> TotalPower/11
  statusDispatchPwr/1 -> TotalPower/13
  Supervisor/1 -> Trm33/1
  TotalPower/1 -> out_telemetry/1
  ModeDbl/1 -> telemetry_el2/1

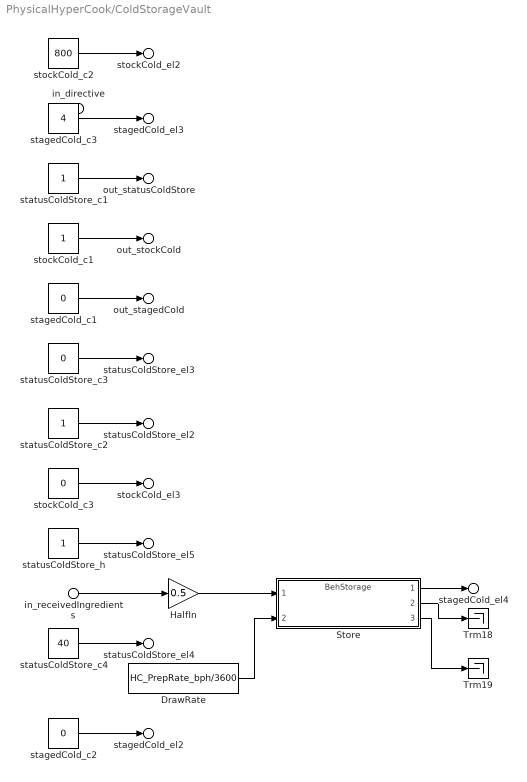
== system PhysicalHyperCook/ColdStorageVault ==
  in_receivedIngredients : Inport  PortName=receivedIngredients  Element=flow_bps
  in_directive : Inport  Port=2  PortName=directive  Element=setpoint
  DrawRate : Constant  Value=HC_PrepRate_bph/3600
  HalfIn : Gain  Gain=0.5
  Store : ModelReference  ModelNameDialog=BehStorage  UsingDefaultArgumentValue=0,0  SimulationMode=Normal  ModelReferenceVersion=1.4
  Trm18 : Terminator
  Trm19 : Terminator
  stagedCold_c1 : Constant  Value=0
  stagedCold_c2 : Constant  Value=0
  stagedCold_c3 : Constant  Value=4
  statusColdStore_c1 : Constant
  statusColdStore_c2 : Constant
  statusColdStore_c3 : Constant  Value=0
  statusColdStore_c4 : Constant  Value=40
  statusColdStore_h : Constant
  stockCold_c1 : Constant
  stockCold_c2 : Constant  Value=800
  stockCold_c3 : Constant  Value=0
  out_stagedCold : Outport  PortName=stagedCold  Element=palletId
  stagedCold_el2 : Outport  PortName=stagedCold  Element=mass_kg
  stagedCold_el3 : Outport  PortName=stagedCold  Element=temp_C
  stagedCold_el4 : Outport  PortName=stagedCold  Element=flow_bps
  out_stockCold : Outport  Port=2  PortName=stockCold  Element=itemId
  stockCold_el2 : Outport  Port=2  PortName=stockCold  Element=qty_units
  stockCold_el3 : Outport  Port=2  PortName=stockCold  Element=error_pct
  out_statusColdStore : Outport  Port=3  PortName=statusColdStore  Element=unitId
  statusColdStore_el2 : Outport  Port=3  PortName=statusColdStore  Element=opState
  statusColdStore_el3 : Outport  Port=3  PortName=statusColdStore  Element=faultCode
  statusColdStore_el4 : Outport  Port=3  PortName=statusColdStore  Element=power_kW
  statusColdStore_el5 : Outport  Port=3  PortName=statusColdStore  Element=health
  wires:
  stockCold_c2/1 -> stockCold_el2/1
  statusColdStore_c3/1 -> statusColdStore_el3/1
  stagedCold_c3/1 -> stagedCold_el3/1
  stockCold_c1/1 -> out_stockCold/1
  statusColdStore_c1/1 -> out_statusColdStore/1
  stagedCold_c1/1 -> out_stagedCold/1
  statusColdStore_c2/1 -> statusColdStore_el2/1
  stockCold_c3/1 -> stockCold_el3/1
  statusColdStore_h/1 -> statusColdStore_el5/1
  in_receivedIngredients/1 -> HalfIn/1
  statusColdStore_c4/1 -> statusColdStore_el4/1
  stagedCold_c2/1 -> stagedCold_el2/1
  HalfIn/1 -> Store/1
  DrawRate/1 -> Store/2
  Store/1 -> stagedCold_el4/1
  Store/2 -> Trm18/1
  Store/3 -> Trm19/1

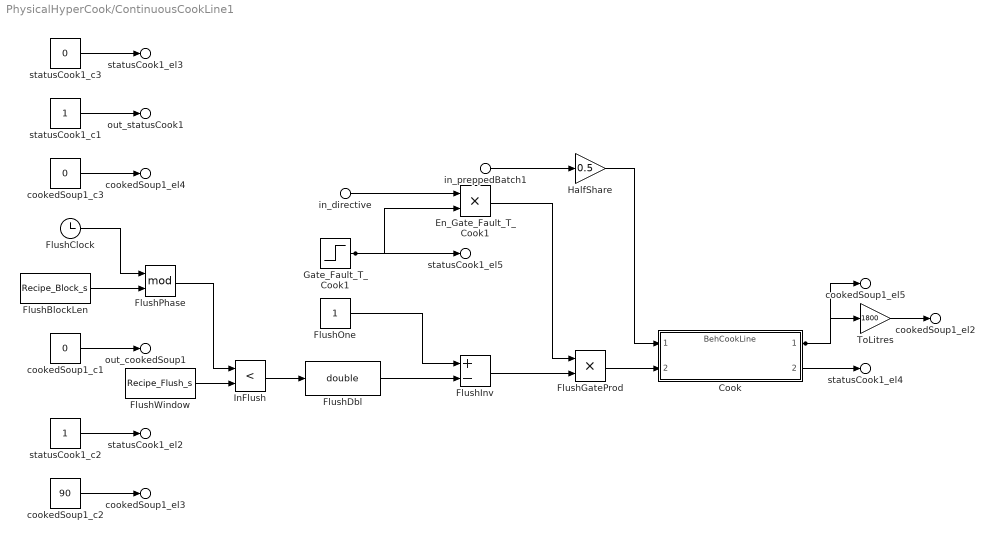
== system PhysicalHyperCook/ContinuousCookLine1 ==
  in_preppedBatch1 : Inport  PortName=preppedBatch1  Element=flow_bps
  in_directive : Inport  Port=2  PortName=directive  Element=setpoint
  Cook : ModelReference  ModelNameDialog=BehCookLine  UsingDefaultArgumentValue=0,0,0,0  SimulationMode=Normal  ModelReferenceVersion=1.4
  En_Gate_Fault_T_Cook1 : Product
  FlushBlockLen : Constant  Value=Recipe_Block_s
  FlushClock : Clock
  FlushDbl : DataTypeConversion  OutDataTypeStr=double  SaturateOnIntegerOverflow=off  RndMeth=Floor
  FlushGateProd : Product
  FlushInv : Sum  Inputs=+-
  FlushOne : Constant
  FlushPhase : Math  Operator=mod
  FlushWindow : Constant  Value=Recipe_Flush_s
  Gate_Fault_T_Cook1 : Step  Time=Fault_T_Cook1  InitialValue=1  FinalValue=0  SampleTime=0
  HalfShare : Gain  Gain=0.5
  InFlush : RelationalOperator  Operator=<  OutDataTypeStr=boolean  RndMeth=Simplest  InputSameDT=off
  ToLitres : Gain  Gain=1800
  cookedSoup1_c1 : Constant  Value=0
  cookedSoup1_c2 : Constant  Value=90
  cookedSoup1_c3 : Constant  Value=0
  statusCook1_c1 : Constant
  statusCook1_c2 : Constant
  statusCook1_c3 : Constant  Value=0
  out_cookedSoup1 : Outport  PortName=cookedSoup1  Element=batchId
  cookedSoup1_el2 : Outport  PortName=cookedSoup1  Element=volume_L
  cookedSoup1_el3 : Outport  PortName=cookedSoup1  Element=temp_C
  cookedSoup1_el4 : Outport  PortName=cookedSoup1  Element=contamination_ppm
  cookedSoup1_el5 : Outport  PortName=cookedSoup1  Element=flow_bps
  out_statusCook1 : Outport  Port=2  PortName=statusCook1  Element=unitId
  statusCook1_el2 : Outport  Port=2  PortName=statusCook1  Element=opState
  statusCook1_el3 : Outport  Port=2  PortName=statusCook1  Element=faultCode
  statusCook1_el4 : Outport  Port=2  PortName=statusCook1  Element=power_kW
  statusCook1_el5 : Outport  Port=2  PortName=statusCook1  Element=health
  wires:
  cookedSoup1_c1/1 -> out_cookedSoup1/1
  Cook/1 -> cookedSoup1_el5/1, ToLitres/1
  statusCook1_c3/1 -> statusCook1_el3/1
  statusCook1_c1/1 -> out_statusCook1/1
  cookedSoup1_c3/1 -> cookedSoup1_el4/1
  HalfShare/1 -> Cook/1
  FlushClock/1 -> FlushPhase/1
  statusCook1_c2/1 -> statusCook1_el2/1
  FlushBlockLen/1 -> FlushPhase/2
  cookedSoup1_c2/1 -> cookedSoup1_el3/1
  FlushPhase/1 -> InFlush/1
  in_directive/1 -> En_Gate_Fault_T_Cook1/1
  FlushWindow/1 -> InFlush/2
  Cook/2 -> statusCook1_el4/1
  InFlush/1 -> FlushDbl/1
  Gate_Fault_T_Cook1/1 -> En_Gate_Fault_T_Cook1/2, statusCook1_el5/1
  FlushOne/1 -> FlushInv/1
  FlushDbl/1 -> FlushInv/2
  in_preppedBatch1/1 -> HalfShare/1
  En_Gate_Fault_T_Cook1/1 -> FlushGateProd/1
  FlushInv/1 -> FlushGateProd/2
  FlushGateProd/1 -> Cook/2
  ToLitres/1 -> cookedSoup1_el2/1

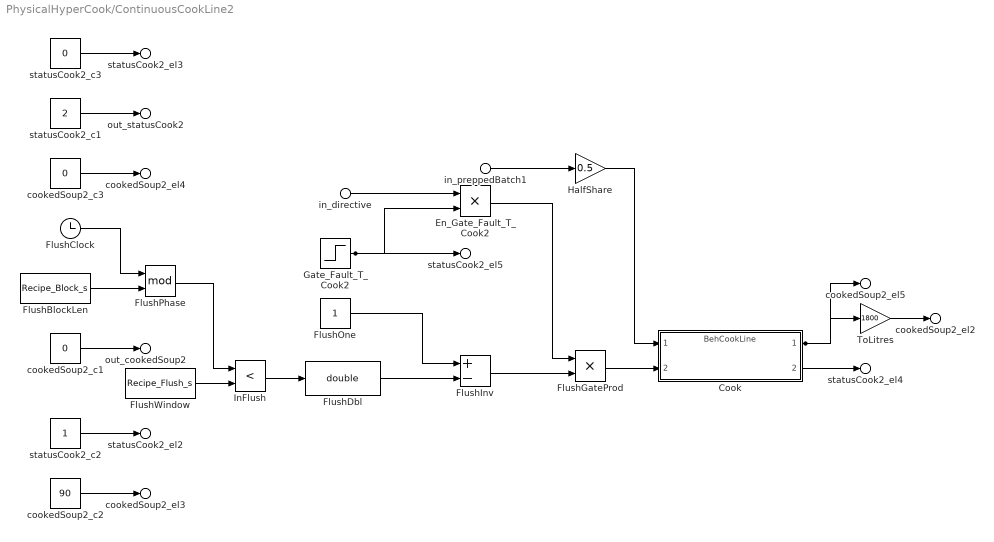
== system PhysicalHyperCook/ContinuousCookLine2 ==
  in_preppedBatch1 : Inport  PortName=preppedBatch1  Element=flow_bps
  in_directive : Inport  Port=2  PortName=directive  Element=setpoint
  Cook : ModelReference  ModelNameDialog=BehCookLine  UsingDefaultArgumentValue=0,0,0,0  SimulationMode=Normal  ModelReferenceVersion=1.4
  En_Gate_Fault_T_Cook2 : Product
  FlushBlockLen : Constant  Value=Recipe_Block_s
  FlushClock : Clock
  FlushDbl : DataTypeConversion  OutDataTypeStr=double  SaturateOnIntegerOverflow=off  RndMeth=Floor
  FlushGateProd : Product
  FlushInv : Sum  Inputs=+-
  FlushOne : Constant
  FlushPhase : Math  Operator=mod
  FlushWindow : Constant  Value=Recipe_Flush_s
  Gate_Fault_T_Cook2 : Step  Time=Fault_T_Cook2  InitialValue=1  FinalValue=0  SampleTime=0
  HalfShare : Gain  Gain=0.5
  InFlush : RelationalOperator  Operator=<  OutDataTypeStr=boolean  RndMeth=Simplest  InputSameDT=off
  ToLitres : Gain  Gain=1800
  cookedSoup2_c1 : Constant  Value=0
  cookedSoup2_c2 : Constant  Value=90
  cookedSoup2_c3 : Constant  Value=0
  statusCook2_c1 : Constant  Value=2
  statusCook2_c2 : Constant
  statusCook2_c3 : Constant  Value=0
  out_cookedSoup2 : Outport  PortName=cookedSoup2  Element=batchId
  cookedSoup2_el2 : Outport  PortName=cookedSoup2  Element=volume_L
  cookedSoup2_el3 : Outport  PortName=cookedSoup2  Element=temp_C
  cookedSoup2_el4 : Outport  PortName=cookedSoup2  Element=contamination_ppm
  cookedSoup2_el5 : Outport  PortName=cookedSoup2  Element=flow_bps
  out_statusCook2 : Outport  Port=2  PortName=statusCook2  Element=unitId
  statusCook2_el2 : Outport  Port=2  PortName=statusCook2  Element=opState
  statusCook2_el3 : Outport  Port=2  PortName=statusCook2  Element=faultCode
  statusCook2_el4 : Outport  Port=2  PortName=statusCook2  Element=power_kW
  statusCook2_el5 : Outport  Port=2  PortName=statusCook2  Element=health
  wires:
  statusCook2_c3/1 -> statusCook2_el3/1
  cookedSoup2_c2/1 -> cookedSoup2_el3/1
  statusCook2_c1/1 -> out_statusCook2/1
  Cook/2 -> statusCook2_el4/1
  cookedSoup2_c1/1 -> out_cookedSoup2/1
  cookedSoup2_c3/1 -> cookedSoup2_el4/1
  in_directive/1 -> En_Gate_Fault_T_Cook2/1
  FlushClock/1 -> FlushPhase/1
  FlushBlockLen/1 -> FlushPhase/2
  statusCook2_c2/1 -> statusCook2_el2/1
  in_preppedBatch1/1 -> HalfShare/1
  FlushPhase/1 -> InFlush/1
  FlushWindow/1 -> InFlush/2
  Gate_Fault_T_Cook2/1 -> En_Gate_Fault_T_Cook2/2, statusCook2_el5/1
  InFlush/1 -> FlushDbl/1
  FlushOne/1 -> FlushInv/1
  FlushInv/1 -> FlushGateProd/2
  FlushDbl/1 -> FlushInv/2
  En_Gate_Fault_T_Cook2/1 -> FlushGateProd/1
  HalfShare/1 -> Cook/1
  FlushGateProd/1 -> Cook/2
  Cook/1 -> cookedSoup2_el5/1, ToLitres/1
  ToLitres/1 -> cookedSoup2_el2/1

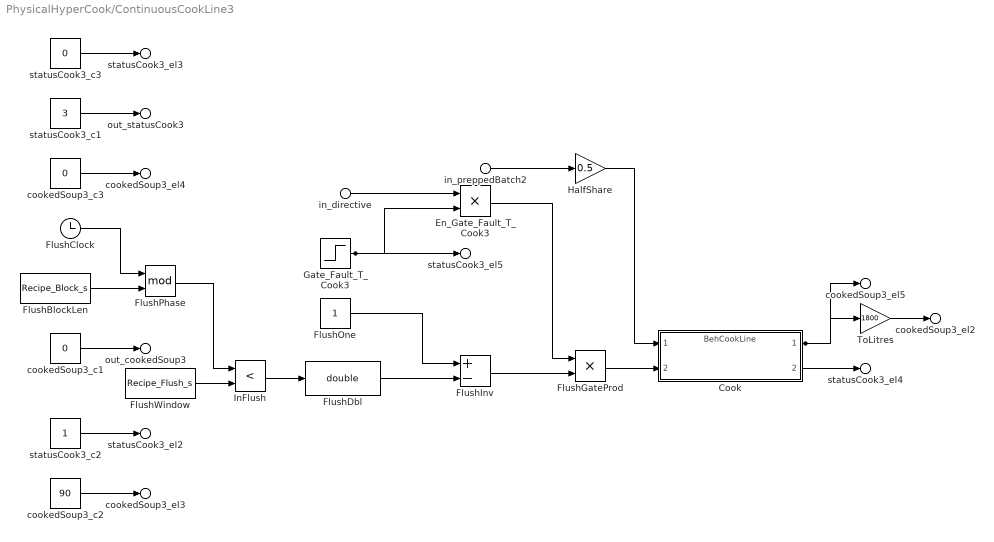
== system PhysicalHyperCook/ContinuousCookLine3 ==
  in_preppedBatch2 : Inport  PortName=preppedBatch2  Element=flow_bps
  in_directive : Inport  Port=2  PortName=directive  Element=setpoint
  Cook : ModelReference  ModelNameDialog=BehCookLine  UsingDefaultArgumentValue=0,0,0,0  SimulationMode=Normal  ModelReferenceVersion=1.4
  En_Gate_Fault_T_Cook3 : Product
  FlushBlockLen : Constant  Value=Recipe_Block_s
  FlushClock : Clock
  FlushDbl : DataTypeConversion  OutDataTypeStr=double  SaturateOnIntegerOverflow=off  RndMeth=Floor
  FlushGateProd : Product
  FlushInv : Sum  Inputs=+-
  FlushOne : Constant
  FlushPhase : Math  Operator=mod
  FlushWindow : Constant  Value=Recipe_Flush_s
  Gate_Fault_T_Cook3 : Step  Time=Fault_T_Cook3  InitialValue=1  FinalValue=0  SampleTime=0
  HalfShare : Gain  Gain=0.5
  InFlush : RelationalOperator  Operator=<  OutDataTypeStr=boolean  RndMeth=Simplest  InputSameDT=off
  ToLitres : Gain  Gain=1800
  cookedSoup3_c1 : Constant  Value=0
  cookedSoup3_c2 : Constant  Value=90
  cookedSoup3_c3 : Constant  Value=0
  statusCook3_c1 : Constant  Value=3
  statusCook3_c2 : Constant
  statusCook3_c3 : Constant  Value=0
  out_cookedSoup3 : Outport  PortName=cookedSoup3  Element=batchId
  cookedSoup3_el2 : Outport  PortName=cookedSoup3  Element=volume_L
  cookedSoup3_el3 : Outport  PortName=cookedSoup3  Element=temp_C
  cookedSoup3_el4 : Outport  PortName=cookedSoup3  Element=contamination_ppm
  cookedSoup3_el5 : Outport  PortName=cookedSoup3  Element=flow_bps
  out_statusCook3 : Outport  Port=2  PortName=statusCook3  Element=unitId
  statusCook3_el2 : Outport  Port=2  PortName=statusCook3  Element=opState
  statusCook3_el3 : Outport  Port=2  PortName=statusCook3  Element=faultCode
  statusCook3_el4 : Outport  Port=2  PortName=statusCook3  Element=power_kW
  statusCook3_el5 : Outport  Port=2  PortName=statusCook3  Element=health
  wires:
  FlushClock/1 -> FlushPhase/1
  statusCook3_c3/1 -> statusCook3_el3/1
  statusCook3_c1/1 -> out_statusCook3/1
  cookedSoup3_c2/1 -> cookedSoup3_el3/1
  ToLitres/1 -> cookedSoup3_el2/1
  En_Gate_Fault_T_Cook3/1 -> FlushGateProd/1
  FlushBlockLen/1 -> FlushPhase/2
  cookedSoup3_c3/1 -> cookedSoup3_el4/1
  FlushDbl/1 -> FlushInv/2
  cookedSoup3_c1/1 -> out_cookedSoup3/1
  in_preppedBatch2/1 -> HalfShare/1
  FlushOne/1 -> FlushInv/1
  statusCook3_c2/1 -> statusCook3_el2/1
  FlushPhase/1 -> InFlush/1
  FlushWindow/1 -> InFlush/2
  InFlush/1 -> FlushDbl/1
  in_directive/1 -> En_Gate_Fault_T_Cook3/1
  Gate_Fault_T_Cook3/1 -> En_Gate_Fault_T_Cook3/2, statusCook3_el5/1
  FlushInv/1 -> FlushGateProd/2
  HalfShare/1 -> Cook/1
  FlushGateProd/1 -> Cook/2
  Cook/1 -> ToLitres/1, cookedSoup3_el5/1
  Cook/2 -> statusCook3_el4/1

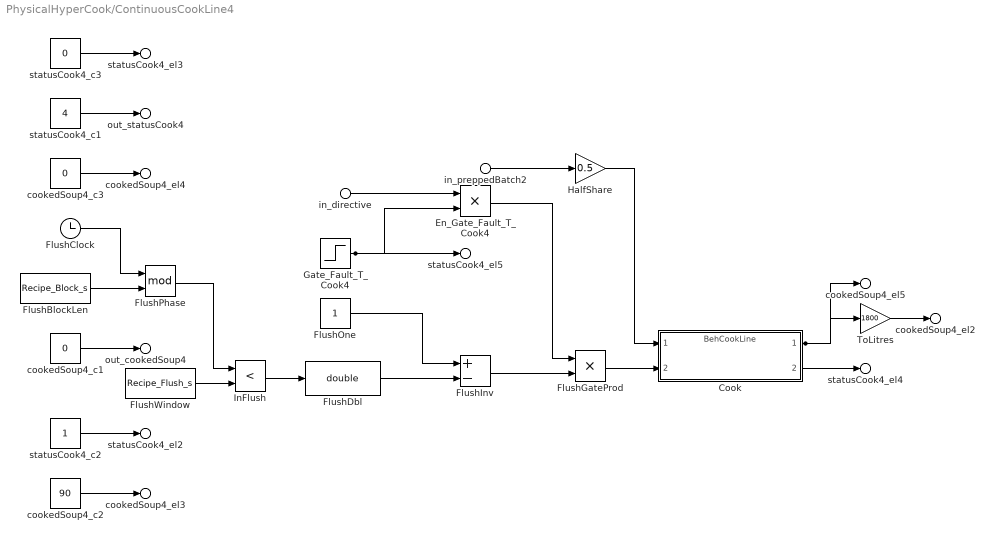
== system PhysicalHyperCook/ContinuousCookLine4 ==
  in_preppedBatch2 : Inport  PortName=preppedBatch2  Element=flow_bps
  in_directive : Inport  Port=2  PortName=directive  Element=setpoint
  Cook : ModelReference  ModelNameDialog=BehCookLine  UsingDefaultArgumentValue=0,0,0,0  SimulationMode=Normal  ModelReferenceVersion=1.4
  En_Gate_Fault_T_Cook4 : Product
  FlushBlockLen : Constant  Value=Recipe_Block_s
  FlushClock : Clock
  FlushDbl : DataTypeConversion  OutDataTypeStr=double  SaturateOnIntegerOverflow=off  RndMeth=Floor
  FlushGateProd : Product
  FlushInv : Sum  Inputs=+-
  FlushOne : Constant
  FlushPhase : Math  Operator=mod
  FlushWindow : Constant  Value=Recipe_Flush_s
  Gate_Fault_T_Cook4 : Step  Time=Fault_T_Cook4  InitialValue=1  FinalValue=0  SampleTime=0
  HalfShare : Gain  Gain=0.5
  InFlush : RelationalOperator  Operator=<  OutDataTypeStr=boolean  RndMeth=Simplest  InputSameDT=off
  ToLitres : Gain  Gain=1800
  cookedSoup4_c1 : Constant  Value=0
  cookedSoup4_c2 : Constant  Value=90
  cookedSoup4_c3 : Constant  Value=0
  statusCook4_c1 : Constant  Value=4
  statusCook4_c2 : Constant
  statusCook4_c3 : Constant  Value=0
  out_cookedSoup4 : Outport  PortName=cookedSoup4  Element=batchId
  cookedSoup4_el2 : Outport  PortName=cookedSoup4  Element=volume_L
  cookedSoup4_el3 : Outport  PortName=cookedSoup4  Element=temp_C
  cookedSoup4_el4 : Outport  PortName=cookedSoup4  Element=contamination_ppm
  cookedSoup4_el5 : Outport  PortName=cookedSoup4  Element=flow_bps
  out_statusCook4 : Outport  Port=2  PortName=statusCook4  Element=unitId
  statusCook4_el2 : Outport  Port=2  PortName=statusCook4  Element=opState
  statusCook4_el3 : Outport  Port=2  PortName=statusCook4  Element=faultCode
  statusCook4_el4 : Outport  Port=2  PortName=statusCook4  Element=power_kW
  statusCook4_el5 : Outport  Port=2  PortName=statusCook4  Element=health
  wires:
  cookedSoup4_c1/1 -> out_cookedSoup4/1
  FlushDbl/1 -> FlushInv/2
  FlushClock/1 -> FlushPhase/1
  FlushGateProd/1 -> Cook/2
  statusCook4_c3/1 -> statusCook4_el3/1
  HalfShare/1 -> Cook/1
  statusCook4_c1/1 -> out_statusCook4/1
  statusCook4_c2/1 -> statusCook4_el2/1
  cookedSoup4_c3/1 -> cookedSoup4_el4/1
  FlushBlockLen/1 -> FlushPhase/2
  cookedSoup4_c2/1 -> cookedSoup4_el3/1
  FlushPhase/1 -> InFlush/1
  FlushWindow/1 -> InFlush/2
  InFlush/1 -> FlushDbl/1
  in_directive/1 -> En_Gate_Fault_T_Cook4/1
  Gate_Fault_T_Cook4/1 -> En_Gate_Fault_T_Cook4/2, statusCook4_el5/1
  FlushOne/1 -> FlushInv/1
  in_preppedBatch2/1 -> HalfShare/1
  En_Gate_Fault_T_Cook4/1 -> FlushGateProd/1
  FlushInv/1 -> FlushGateProd/2
  Cook/1 -> ToLitres/1, cookedSoup4_el5/1
  Cook/2 -> statusCook4_el4/1
  ToLitres/1 -> cookedSoup4_el2/1

== system PhysicalHyperCook/ConveyorNetwork ==
  in_transportDirective : Inport  PortName=transportDirective
  statusTransport_c1 : Constant
  statusTransport_c2 : Constant
  statusTransport_c3 : Constant  Value=0
  statusTransport_c4 : Constant  Value=25
  statusTransport_h : Constant
  out_statusTransport : Outport  PortName=statusTransport  Element=unitId
  statusTransport_el2 : Outport  PortName=statusTransport  Element=opState
  statusTransport_el3 : Outport  PortName=statusTransport  Element=faultCode
  statusTransport_el4 : Outport  PortName=statusTransport  Element=power_kW
  statusTransport_el5 : Outport  PortName=statusTransport  Element=health
  wires:
  statusTransport_h/1 -> statusTransport_el5/1
  statusTransport_c1/1 -> out_statusTransport/1
  statusTransport_c2/1 -> statusTransport_el2/1
  statusTransport_c3/1 -> statusTransport_el3/1
  statusTransport_c4/1 -> statusTransport_el4/1

== system PhysicalHyperCook/FusionPowerPlant ==
  in_directive : Inport  PortName=directive
  statusPower_c1 : Constant
  statusPower_c2 : Constant
  statusPower_c3 : Constant  Value=0
  statusPower_c4 : Constant  Value=0
  statusPower_h : Constant
  out_statusPower : Outport  PortName=statusPower  Element=unitId
  statusPower_el2 : Outport  PortName=statusPower  Element=opState
  statusPower_el3 : Outport  PortName=statusPower  Element=faultCode
  statusPower_el4 : Outport  PortName=statusPower  Element=power_kW
  statusPower_el5 : Outport  PortName=statusPower  Element=health
  wires:
  statusPower_c4/1 -> statusPower_el4/1
  statusPower_h/1 -> statusPower_el5/1
  statusPower_c3/1 -> statusPower_el3/1
  statusPower_c1/1 -> out_statusPower/1
  statusPower_c2/1 -> statusPower_el2/1

== system PhysicalHyperCook/GravityCompensatorArray ==
  in_ambientGravity : Inport  PortName=ambientGravity  Element=gravity_g
  envStatus_c1 : Constant  Value=100
  out_envStatus : Outport  PortName=envStatus  Element=gravity_g
  envStatus_el2 : Outport  PortName=envStatus  Element=compensation_pct
  wires:
  in_ambientGravity/1 -> out_envStatus/1  "ambientGravity"
  envStatus_c1/1 -> envStatus_el2/1

== system PhysicalHyperCook/HighSpeedPackagingLine ==
  in_approvedSoup : Inport  PortName=approvedSoup  Element=flow_bps
  in_directive : Inport  Port=2  PortName=directive  Element=setpoint
  En_Gate_Fault_T_Pack : Product
  Gate_Fault_T_Pack : Step  Time=Fault_T_Pack  InitialValue=1  FinalValue=0  SampleTime=0
  Pack : ModelReference  ModelNameDialog=BehPackager  UsingDefaultArgumentValue=0,0  SimulationMode=Normal  ModelReferenceVersion=1.5
  PackDraw : Constant  Value=HC_PackRate_bph/3600
  Surge : ModelReference  ModelNameDialog=BehStorage  UsingDefaultArgumentValue=0,0  SimulationMode=Normal  ModelReferenceVersion=1.4
  Trm30 : Terminator
  Trm31 : Terminator
  sealedContainers_c1 : Constant  Value=0
  sealedContainers_c2 : Constant  Value=0
  sealedContainers_c3 : Constant  Value=365
  statusPack_c1 : Constant
  statusPack_c2 : Constant
  statusPack_c3 : Constant  Value=0
  statusPack_c4 : Constant  Value=35
  out_sealedContainers : Outport  PortName=sealedContainers  Element=batchId
  sealedContainers_el2 : Outport  PortName=sealedContainers  Element=count
  sealedContainers_el3 : Outport  PortName=sealedContainers  Element=sealRating_days
  sealedContainers_el4 : Outport  PortName=sealedContainers  Element=flow_bps
  out_statusPack : Outport  Port=2  PortName=statusPack  Element=unitId
  statusPack_el2 : Outport  Port=2  PortName=statusPack  Element=opState
  statusPack_el3 : Outport  Port=2  PortName=statusPack  Element=faultCode
  statusPack_el4 : Outport  Port=2  PortName=statusPack  Element=power_kW
  statusPack_el5 : Outport  Port=2  PortName=statusPack  Element=health
  wires:
  statusPack_c2/1 -> statusPack_el2/1
  in_directive/1 -> En_Gate_Fault_T_Pack/1
  sealedContainers_c3/1 -> sealedContainers_el3/1
  sealedContainers_c1/1 -> out_sealedContainers/1
  statusPack_c4/1 -> statusPack_el4/1
  Surge/1 -> Pack/1
  Gate_Fault_T_Pack/1 -> En_Gate_Fault_T_Pack/2, statusPack_el5/1
  statusPack_c1/1 -> out_statusPack/1
  statusPack_c3/1 -> statusPack_el3/1
  in_approvedSoup/1 -> Surge/1
  PackDraw/1 -> Surge/2
  sealedContainers_c2/1 -> sealedContainers_el2/1
  Surge/2 -> Trm30/1
  En_Gate_Fault_T_Pack/1 -> Pack/2
  Surge/3 -> Trm31/1
  Pack/1 -> sealedContainers_el4/1
